simulink model "GoHomeController"  (R2016a)
settings: Solver=ode5  StartTime=0.0  StopTime=100  FixedStep=1/100  RelTol=1e-3  AbsTol=1e-6
model workspace: external: MAT-File GoHomeWorkspace1.mat (data not in the file)
values from neighbouring files (symbols this model uses):
  filtDen = [1 -2.5774735647 5.16845279747 -6.83689517845 7.38438625477 -6.22361169904 4.37103521312 -2.50318155423 1.19677078786 -0.46926551656 0.151337698262 -0.0392326536536 ... (17 elements, 1x17)]    [GoHomeWorkspace.mat]
  filtNum = [9.60149042661e-06 0.000153623846826 0.00115217885119 0.0053768346389 0.0174747125764 0.0419393101834 0.0768887353363 0.10984105048 0.12357118179 0.10984105048 0.0768887353363 0.0419393101834 ... (17 elements, 1x17)]    [GoHomeWorkspace.mat]
  K = [0.865125 0 0 0 0 0.87025 0 0 8 0 0 0 ... (20 elements, 2x10)]    [GoHomeWorkspace.mat]
  Ts = 0.01    [GoHomeWorkspace.mat]
undefined symbols (not defined in the file or in its folder): Crane3D_RangeBit, Crane3D_ScaleCoeff, DiscIntNeverNeededParam
undefined symbols (not defined in the file): RTDAC4PCIBaseAddress
libraries: simulink x1
(part 1 of 11)
settings Model: SimulationMode=external  ExtModeTrigDuration=12000  ExtModeTrigLevel=0.400000  Creator=jims  LastModifiedBy=im1716
settings SolverCC: AutoInsertRateTranBlk=on  InsertRTBMode=Never (minimum delay)
settings DataIOCC: ExternalInput=[]  InitialState=[]  MaxDataPoints=5000  SaveFormat=StructureWithTime  SignalLoggingSaveFormat=ModelDataLogs
settings OptimizationCC: BooleanDataType=off  ExpressionDepthLimit=2147483647  InitFltsAndDblsToZero=on
settings DebuggingCC: SaveWithParameterizedLinksMsg=none  UnderspecifiedInitializationDetection=Classic  MergeDetectMultiDrivingBlocksExec=none  SignalResolutionControl=TryResolveAllWithWarning  MultiTaskDSMMsg=warning  MultiTaskCondExecSysMsg=none  IntegerOverflowMsg=none  FcnCallInpInsideContextMsg=EnableAllAsWarning  AllowSymbolicDim=off  StateNameClashWarn=warning  IntegerSaturationMsg=none
settings HardwareCC: ProdBitPerLong=64  ProdLargestAtomicFloat=None  ProdHWDeviceType=Intel->x86-64  TargetBitPerLong=64  TargetBitPerPointer=64  TargetIntDivRoundTo=Zero  TargetEndianess=LittleEndian  TargetWordSize=64  TargetHWDeviceType=Intel->x86-64
settings ModelReferenceCC: UpdateModelReferenceTargets=Force  PropagateSignalLabelsOutOfModel=off
settings RTWCC: SystemTargetFile=sldrt.tlc  TemplateMakefile=sldrt.tmf  Description=Simulink Desktop Real-Time  RTWCompilerOptimization=on
settings CodeAppCC: MaxIdLength=95
settings TargetCC: TargetFcnLib=ansi_tfl_tmw.mat  TargetPreCompLibLocation=c:\matlab\R2016a\toolbox\sldrt\lib\win64  ModelReferenceCompliant=off  CompOptLevelCompliant=off  GeneratePreprocessorConditionals=Use local settings
settings ConfigComp: CovSFcnEnable=off

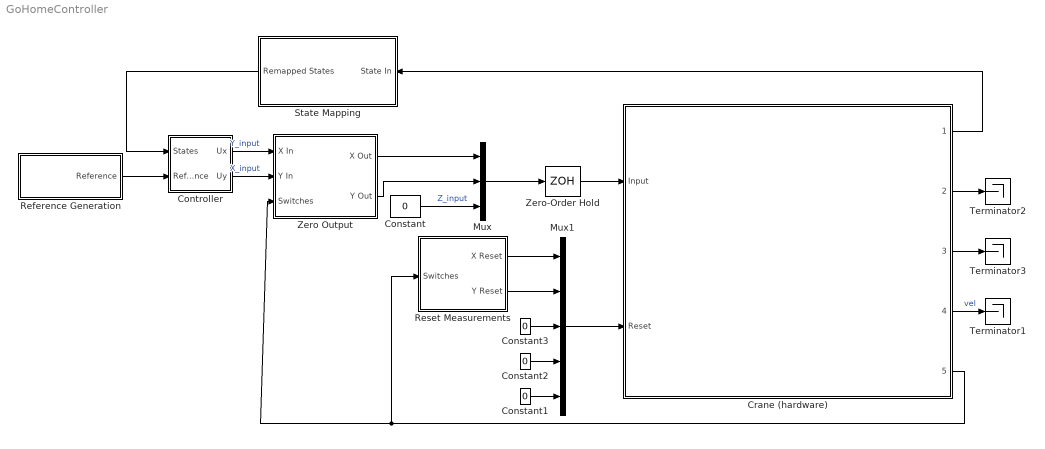
== system GoHomeController ==
  Constant{,1..3} (4 alike) : Constant  Value=0
  Controller : Subsystem
  Crane (hardware) : Subsystem
      mask Display:
